simulink model "SI_2_simulink"  (R2020b)
settings: Solver=FixedStepAuto  StartTime=0.0  StopTime=20.0  FixedStep=0.01  MaxStep=0.01  RelTol=1e-2  AbsTol=1e-2  EnableMultiTasking=on
undefined symbols (not defined in the file): b
libraries: pid_lib x1
settings Model: Creator=jerem  LastModifiedBy=jerem
settings OptimizationCC: DenormalBehavior=FlushToZero

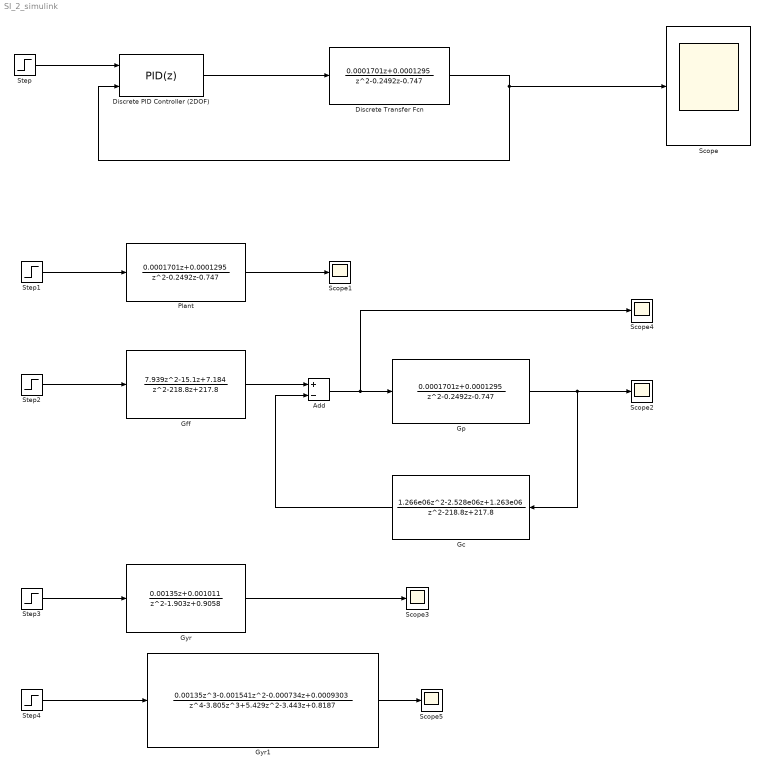
== system SI_2_simulink ==
  Add : Sum  Inputs=+-
  Discrete Transfer Fcn : DiscreteTransferFcn  Numerator=[0.0001701, 0.0001295]  Denominator=[1, -0.2492, -0.747]  SampleTime=0.01
  Discrete PID Controller (2DOF) : pid_lib/PID Controller (2DOF)  Controller=PID  Form=Parallel  TimeDomain=Discrete-time  UseExternalTs=off  SampleTime=-1  IntegratorMethod=Forward Euler  FilterMethod=Forward Euler  ControllerParametersSource=internal  P=-12.8474  I=-0.0087  D=-58.3677  UseFilter=on  N=-2.1683e+04  b=b  c=c  TunerSelectOption=Transfer Function Based (PID Tuner App)  InitialConditionSource=internal  InitialConditionForIntegrator=0  InitialConditionForFilter=0  DifferentiatorICPrevScaledInput=0  ExternalReset=none  TrackingMode=off  Kt=1  LimitOutput=off  SatLimitsSource=internal  UpperSaturationLimit=inf  LowerSaturationLimit=-inf  LinearizeAsGain=off  AntiWindupMode=none  Kb=1  POutMin=[]  POutMax=[]  IOutMin=[]  IOutMax=[]  DOutMin=[]  DOutMax=[]  NOutMin=[]  NOutMax=[]  bOutMin=[]  bOutMax=[]  cOutMin=[]  cOutMax=[]  SumOutMin=[]  SumOutMax=[]  SaturationOutMin=[]  SaturationOutMax=[]  PParamMin=[]  PParamMax=[]  IParamMin=[]  IParamMax=[]  DParamMin=[]  DParamMax=[]  NParamMin=[]  NParamMax=[]  bParamMin=[]  bParamMax=[]  cParamMin=[]  cParamMax=[]  KbParamMin=[]  KbParamMax=[]  KtParamMin=[]  KtParamMax=[]  KbOutMin=[]  KbOutMax=[]  KtOutMin=[]  KtOutMax=[]  IntegratorOutMin=[]  IntegratorOutMax=[]  FilterOutMin=[]  FilterOutMax=[]  SumI1OutMin=[]  SumI1OutMax=[]  SumI2OutMin=[]  SumI2OutMax=[]  SumI3OutMin=[]  SumI3OutMax=[]  SumI4OutMin=[]  SumI4OutMax=[]  SumDOutMin=[]  SumDOutMax=[]  Sum1OutMin=[]  Sum1OutMax=[]  Sum2OutMin=[]  Sum2OutMax=[]  Sum3OutMin=[]  Sum3OutMax=[]  DifferentiatorOutMin=[]  DifferentiatorOutMax=[]  FilterDiffOutCoefMin=[]  FilterDiffOutCoefMax=[]  ReciprocalOutMin=[]  ReciprocalOutMax=[]  SumDenOutMin=[]  SumDenOutMax=[]  SumNumOutMin=[]  SumNumOutMax=[]  DivideOutMin=[]  DivideOutMax=[]  UdiffTsProdOutMin=[]  UdiffTsProdOutMax=[]  NTsProdOutMin=[]  NTsProdOutMax=[]  UintegralTsProdOutMin=[]  UintegralTsProdOutMax=[]  UngainTsProdOutMin=[]  UngainTsProdOutMax=[]  IntegratorContinuousStateAttributes=''  IntegratorStateMustResolveToSignalObject=off  IntegratorRTWStateStorageClass=Auto  FilterContinuousStateAttributes=''  FilterStateMustResolveToSignalObject=off  FilterRTWStateStorageClass=Auto  ParallelPVariant=InternalParameters  IdealPVariant=Disabled  IVariant=InternalParameters  DVariant=InternalParameters  bVariant=InternalParameters  cVariant=InternalParameters  IntegratorVariant=Discrete  SatVariant=Disabled  AWVariant=Passthrough  PCopyVariant=Disabled  TRVariant=Disabled  FdbkBlocksVariant=Forward  IdealPFdbkVariant=Disabled  SatFdbkVariant=Disabled  DerivativeFilterVariant=ForwardEulerFilter  NVariant=InternalParameters  NCopyVariant=Disabled  FilterICVariant=InternalICsFilter  IntegratorICVariant=InternalICs  ExternalResetVariant=Disabled  TRSumVariant=Passthrough  SumFdbkVariant=Disabled  SumVariant=Sum_PID  TsampFilterVariant=InternalTs  TsampNgainVariant=Passthrough  TsampIntegralVariant=Passthrough  ExternalSaturationOutDataTypeStr=Inherit: Same as second input
      settings: SourceProductBaseCode=SL
  Gc : DiscreteTransferFcn  Numerator=[1.266e06, -2.528e06, 1.263e06]  Denominator=[1, -218.8, 217.8]  SampleTime=0.01
  Gff : DiscreteTransferFcn  Numerator=[7.939, -15.1, 7.184]  Denominator=[1, -218.8, 217.8]  SampleTime=0.01
  Gp : DiscreteTransferFcn  Numerator=[0.0001701, 0.0001295]  Denominator=[1, -0.2492, -0.747]  SampleTime=0.01
  Gyr : DiscreteTransferFcn  Numerator=[0.00135, 0.001011]  Denominator=[1, -1.903, 0.9058]  SampleTime=0.01
  Gyr1 : DiscreteTransferFcn  Numerator=[0.00135, -0.001541, -0.000734, 0.0009303]  Denominator=[1, -3.805, 5.429, -3.443, 0.8187]  SampleTime=0.01
  Plant : DiscreteTransferFcn  Numerator=[0.0001701, 0.0001295]  Denominator=[1, -0.2492, -0.747]  SampleTime=0.01
  Scope : Scope  NumInputPorts=3
  Scope{1..5} (5 alike) : Scope
  Step : Step  SampleTime=0
  Step1 : Step  SampleTime=0
  Step2 : Step  SampleTime=0.01
  Step3 : Step  SampleTime=0.01
  Step4 : Step  SampleTime=0.01
  wires:
  Discrete Transfer Fcn/1 -> Scope/2, Discrete PID Controller (2DOF)/2
  Step/1 -> Discrete PID Controller (2DOF)/1
  Step1/1 -> Plant/1
  Plant/1 -> Scope1/1
  Step2/1 -> Gff/1
  Gp/1 -> Gc/1, Scope2/1
  Gff/1 -> Add/1
  Add/1 -> Scope4/1, Gp/1
  Gc/1 -> Add/2
  Step3/1 -> Gyr/1
  Gyr/1 -> Scope3/1
  Discrete PID Controller (2DOF)/1 -> Discrete Transfer Fcn/1
  Step4/1 -> Gyr1/1
  Gyr1/1 -> Scope5/1
